simulink model "FlapDuuuuuragControlSimulatorForFriends"  (R2024b)
settings: Solver=VariableStepAuto  StartTime=0.0  StopTime=20  RelTol=1e-3
undefined symbols (not defined in the file): Asymptote, Body_Diameter, Body_Length, csv, DiscIntNeverNeededParam, Dragx, Dragy, Dry_Mass, Empty_Motor_Mass, Fin_Area, Flap_Length, Flap_width, flaps, Integral, Integral_Motor_Curve, Motorx, Motory, num_Flaps, optimize, Pressure, Propellent_Mass, Proportional, Rail_Angle, Temp, time_at_final, time_constants_to_final, wind_direction, wind_speed, wind_Z, Y_int_offset
libraries: simulink x4, simulink_extras x3, slpidlib x2, aerolibwind2 x2, aerolibutil x1, sharedtransform x1, eeGeneralControl x1
(part 1 of 2)
settings Model: PacingRate=10  Creator=jonse  LastModifiedBy=rjsoc
settings RTWCC: GPUComputeCapability=3.5

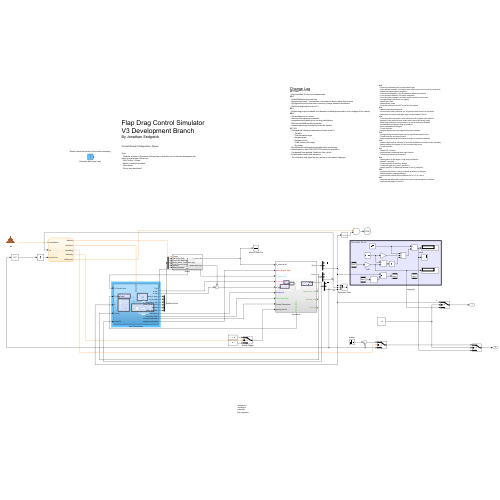
[thumbnail: Simulink's stored preview of the top-level diagram]
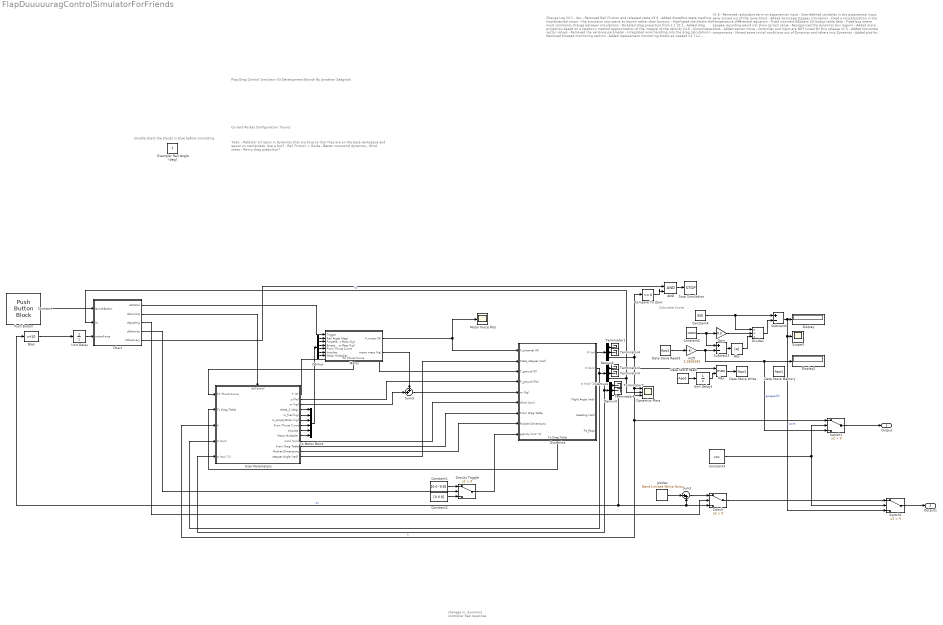
== system FlapDuuuuuragControlSimulatorForFriends ==
  note: changes in:
      |  dynamics
      | controller
      | flap response
  note: Todo:
      |  - Refactor all items in Dynamics that are blue so that they are on the base workspace and easier to manipulate. Use a bus?
      |  - Rail Friction + Guide
      |  - Better crosswind dynamics
      |  - Wind shear
      |  - Re-try drag prediction?
  note: Current Rocket Configuration: Taurus
  note: Double check the blocks in blue before simulating
  note: Calculate Score
  note: Flap Drag Control Simulator
      | V3 Development Branch
      | By Jonathan Sedgwick
  note: Change Log
      | V3.1 - dev
      | - Removed Rail Friction and releated state
      | V3.0
      | - Added Stateflow state machine
      | - Implemented motor - the simulator now starts at launch rather than burnout
      | - Highligted the blocks that most commonly change between simulations
      | - Disabled drag projection from 2.1
      | V2.1
      | - Added drag projection based on a Newton's method approximation of the integral of the velocity
      | V2.0
      | - Consolidated vector values
      | - Removed the variance parameter
      | - Integrated wind handling into the drag calculations
      | - Removed bloated monitoring section
      | - Added replacement monitoring blocks as needed
      | V1.7-L2
      | - Changed the following parameters to those of the L2
      | - Cd table
      | - Flap saturation angle
      | - Apogee target
      | - Apogee scoring
      | - Initial velocity and height
      | - Dry mass
      | - Re-defined the exponential input with better terminology
      | - Added option to use 2022-2023 CFD results for drag force
      | - Condensed User-defined Conditions into a block
      | - Added questionable wind equations
      | - The simulation now stops as soon as the all runs have hit apogee
  note: V1.6
      | - Removed redundant term on exponential input
      | - User-defined variables in the exponential input were moved out of the ramp block
      | - Added Simscape stepper simulation
      | - Fixed a miscalculation in the Temperature differential equation
      | - Fixed incorrect RASaero Cd lookup table data
      | - Fixed bug where apogee recording would not show correct value
      | - Reorganized the dynamics box (again)
      | - Added more plots
      | - Added sensor noise
      | - Controller and Input are NOT tuned for this release
      | V1.5
      | - Added horizontal components
      | - Moved some initial conditions out of Dynamics and others into Dynamics
      | - Added plot for velocity and flight angle (angle of attack? pitch?)
      | V1.4
      | - Fixed bug where simulation would end before all apogees were reached
      | - Apogee is now stored as max height rather than most recent height
      | - Body drag coefficient is now based on a lookup table from RASaero
      | - Incorperated post-apogee drag calculations
      | - More organizational changes
      | - Tuned controller
      | - Apogee displays are now organized by input condition
      | V1.3
      | - Changed from piecewise linear input to exponential input function
      | - Tuned controller and Input function
      | - Major oragnizational and formatting changes to increase readability
      | V1.2
      | - Added a high and low variance to the initial conditions to simulate motor variability
      | - Added displays for apogee in ft and corrosponding score
      | - Tuned controller
      | V1.1
      | - Added PID controller
      | - Implemented a saturated ramp input function
      | - Tuned input function and controller
      | V1.0
      | - Added effects of flap angle on flap drag contribution
      | - Added P controller
      | - Tuned controller to reach an altitude
      | - Combined graph for h and h_prediction
      | - Added graph for % difference between h and h_prediction
      | V0.2
      | - Implemented phisics 1 energy methods prediction for apogee
      | - Added graph for predicted apogee
      | - Implemented external initial conditions for h0, v0, m, and d
      | V0.1
      | - Implemented differential equations for motion and atmosphere conditions
      | - Implemented graphs of h and a
  AND : Logic  IconShape=distinctive  AllPortsSameDT=off  OutDataTypeStr=boolean
  Abs : Abs  SaturateOnIntegerOverflow=off
  Bias : Bias  Bias=10  SaturateOnIntegerOverflow=off
  Chart : Stateflow chart  TreatAsAtomicUnit=on
  Compare To Zero : simulink/Logic and Bit Operations/Compare To Zero  relop=<=  OutDataTypeStr=boolean
  Constant : Constant  Value=0
  Constant1 : Constant  Value=[0 0 -9.8]
  Constant2 : Constant  Value=[0 0 0]
  Constant3 : Constant  Value=csv
  Constant4 : Constant  Value=350
  Constant5 : Constant  Value=10000
  Data Store Read : DataStoreRead  DataStoreName=Apo1  IndexOptions=Index vector (dialog)  Indices=1  OutputSizes=1
  Data Store Read3 : DataStoreRead  DataStoreName=Apo1  IndexOptions=Index vector (dialog)  Indices=1  OutputSizes=1
  Data Store Write : DataStoreWrite  DataStoreName=Apo1  IndexOptions=Index vector (dialog)  Indices=1  OutputSizes=1
  Data Store Memory : DataStoreMemory  DataStoreName=Apo1  WriteAfterWriteMsg=warning  ShowAdditionalParam=off
  Demux : Demux  Outputs=6
  Demux1 : Demux  Outputs=3
  Demux2 : Demux  Outputs=3
  Demux4 : Demux  Outputs=3
  Display : Display
      settings: Format=bank
  Display2 : Display
      settings: Format=bank
  Divide1 : Product  Inputs=*/*
  Dynamics : Subsystem
      settings: PortSchema="{\"entries\":[{\"content\":{\"sides\":[{\"content\":{\"connectorIds\":[\"In1\",\"In2\",\"In3\",\"In4\",\"In5\",\"In6\",\"In7\",\"In8\",\"In9\"]},\"type\":\"ConnectorPlacement.EquallySpacedRectSide\",\"uuid\":\"61cf24c6-4793-46fb-bba1-f2879032278a\"},{\"content\":{\"connectorIds\":[\"Out1\",\"Out2\",\"Out3\",\"Out4\",\"Out5\",\"Out6\"],\"side\":\"RIGHT\"},\"type\":\"ConnectorPlacement.EquallySpacedRectSide\",\"uuid\":\"d36b1d95-1566-4e4d-8085-05406828bfee\"},{\"content\":{\"side\":\"TOP\"},\"type\":\"ConnectorPlacement.EquallySpacedRectSide\",\"uuid\":\"fa8074a3-9b0c-494d-b168-a3d8dc876f37\"},{\"content\":{\"connectorIds\":[\"Out7\"],\"side\":\"BOTTOM\"},\"type\":\"ConnectorPlacement.EquallySpacedRectSide\",\"uuid\":\"d0ccd591-4c20-4f19-a686-a0802005a38c\"}]},\"type\":\"ConnectorPlacement.EquallySpacedConnector\",\"uuid\":\"5370dd20-9b1c-4f64-993b-f7608f424fd6\"}],\"packageUris\":[\"http://schema.mathworks.com/mf0/Connector/R2020b\"],\"version\":\"1.0\"}"
  Dynamics Plots : Scope  NumInputPorts=3
  Example: Rail Angle (deg) : Constant  Value=7
  Gain : Gain  Gain=0.3
  Gravity Toggle : Switch  Criteria=u2 > Threshold  SaturateOnIntegerOverflow=off  InputSameDT=off
  Jostles : simulink/Sources/Band-Limited White Noise  Cov=[0.1]  Ts=0.1  seed=[23341]
  Max : MinMax  Function=max  Inputs=2  ZeroCross=off
  Motor : Subsystem
      settings: PortSchema="{\"entries\":[{\"content\":{\"sides\":[{\"content\":{\"connectorIds\":[\"In1\",\"In2\",\"In3\",\"In4\",\"In5\",\"In6\",\"In7\"]},\"type\":\"ConnectorPlacement.EquallySpacedRectSide\",\"uuid\":\"6892474e-c13b-4b5d-a78a-550e13a4fcf7\"},{\"content\":{\"connectorIds\":[\"Out1\",\"Out2\"],\"side\":\"RIGHT\"},\"type\":\"ConnectorPlacement.EquallySpacedRectSide\",\"uuid\":\"18cd9a73-be62-415c-a5c9-b5315f96bd44\"},{\"content\":{\"side\":\"TOP\"},\"type\":\"ConnectorPlacement.EquallySpacedRectSide\",\"uuid\":\"19941a30-b527-4a81-9ce0-74fdb4c32049\"},{\"content\":{\"connectorIds\":[\"Out3\"],\"side\":\"BOTTOM\"},\"type\":\"ConnectorPlacement.EquallySpacedRectSide\",\"uuid\":\"d47e24a6-a8af-4693-b00f-f9087fef628a\"}]},\"type\":\"ConnectorPlacement.EquallySpacedConnector\",\"uuid\":\"0b620e34-0fcb-46c3-97c7-1b93d7cb0d0f\"}],\"packageUris\":[\"http://schema.mathworks.com/mf0/Connector/R2020b\"],\"version\":\"1.0\"}"
  Motor Force Plot : Scope
  Push Button : PushButtonBlock  ButtonText=Launch  Icon=Triangle  IconAlignment=Top  IconColor=On  OffValue=0.000000
  Scope3 : Scope
  Stop Simulation : Stop
  Subtract2 : Sum  Inputs=+-
  Subtract3 : Sum  Inputs=+-
  Sum1 : Sum  Inputs=|++
  Sum3 : Sum  Inputs=++|
  Switch : Switch  Criteria=u2 > Threshold  SaturateOnIntegerOverflow=off  InputSameDT=off
  Switch1 : Switch  Criteria=u2 > Threshold  SaturateOnIntegerOverflow=off  InputSameDT=off
  Switch2 : Switch  Criteria=u2 > Threshold  SaturateOnIntegerOverflow=off  InputSameDT=off
  Terminator{1..4,7..8} (6 alike) : Terminator
  To Motor Block : BusCreator  Inputs=6
  Unit Delay : UnitDelay  SampleTime=-1  HasFrameUpgradeWarning=on
  Unit Delay1 : UnitDelay  SampleTime=-1  HasFrameUpgradeWarning=on
  User Parameters : Subsystem
      settings: PortSchema="{\"entries\":[{\"content\":{\"sides\":[{\"content\":{\"connectorIds\":[\"In1\",\"In2\",\"In3\",\"In4\",\"In5\"]},\"type\":\"ConnectorPlacement.EquallySpacedRectSide\",\"uuid\":\"67ceafc0-d2dd-45da-bafe-c1e73a1e832c\"},{\"content\":{\"connectorIds\":[\"Out1\",\"Out2\",\"Out3\",\"Out4\",\"Out5\",\"Out6\",\"Out7\",\"Out8\",\"Out9\",\"Out10\",\"Out11\",\"Out12\",\"Out13\"],\"side\":\"RIGHT\"},\"type\":\"ConnectorPlacement.EquallySpacedRectSide\",\"uuid\":\"fdcb3816-6022-4f62-9865-dec1f25bccbe\"},{\"content\":{\"connectorIds\":[\"In6\"],\"side\":\"TOP\"},\"type\":\"ConnectorPlacement.EquallySpacedRectSide\",\"uuid\":\"c0a2d968-8bba-41a7-998d-7d8e966bd078\"}]},\"type\":\"ConnectorPlacement.EquallySpacedConnector\",\"uuid\":\"e02f46ef-3454-4fc3-b120-1dd0bd81dbda\"}],\"packageUris\":[\"http://schema.mathworks.com/mf0/Connector/R2020b\"],\"version\":\"1.0\"}"
  m2ft : Gain  Gain=3.2808399
  Output : Outport
  Output1 : Outport  Port=2
  wires:
  Chart/1(doMotor) -> Motor/1(Trigger)
  Constant/1 -> Chart/1(launchButton)
  Demux1/2 -> Terminator3/1
  Demux1/1 -> Terminator2/1
  Demux1/3 -> Chart/2(Vz), Dynamics Plots/2  "Vz"
  Demux2/1 -> Terminator1/1
  Demux2/2 -> Terminator4/1
  Dynamics/1(R (m)) -> Demux2/1
  Dynamics/2(V (m/s)) -> User Parameters/4(V (m/s)), Demux1/1
  Chart/2(doControl) -> User Parameters/6(doControl)
  User Parameters/10(wind (m/s)) -> Dynamics/6(Wind (m/s))
  Motor/2(motor mass (kg)) -> Sum3/1
  Sum3/1 -> Dynamics/5(m (kg))
  Constant1/1 -> Gravity Toggle/1
  Chart/4(doGravity) -> Gravity Toggle/2
  Constant2/1 -> Gravity Toggle/3
  Gravity Toggle/1 -> Dynamics/9(gravity (m/s^2))
  Unit Delay/1 -> Chart/3(motorForce)
  Chart/5(inRecovery) -> AND/1
  Compare To Zero/1 -> AND/2
  AND/1 -> Stop Simulation/1
  Subtract3/1 -> Abs/1
  Abs/1 -> Divide1/3
  Constant4/1 -> Subtract2/1, Divide1/1
  Subtract2/1 -> Switch2/3, Scope3/1, Display/1  "score"
  Divide1/1 -> Subtract2/2
  Gain/1 -> Divide1/2
  Constant5/1 -> Subtract3/1, Gain/1
  m2ft/1 -> Switch1/3, Display2/1, Subtract3/2  "apogee(ft)"
  Data Store Read/1 -> Unit Delay1/1
  Max/1 -> Data Store Write/1
  Unit Delay1/1 -> Max/2
  Data Store Read3/1 -> m2ft/1
  Demux2/3 -> Compare To Zero/1, User Parameters/3(h), Switch1/1, Dynamics Plots/1, Max/1  "h"
  Demux4/1 -> Terminator7/1
  Dynamics/3(a (m/s^2)) -> User Parameters/5(a (m/s^2)), Demux4/1
  Demux4/3 -> Bias/1, Sum1/2, Switch/3, Dynamics Plots/3  "az"
  Demux4/2 -> Terminator8/1
  Sum1/1 -> Switch/1
  Chart/3(doJostling) -> Switch/2
  Jostles/1 -> Sum1/1
  Switch/1 -> Switch2/1
  Bias/1 -> Unit Delay/1
  Motor/1(F_motor (N)) -> Dynamics/1(F_external (N)), Motor Force Plot/1
  User Parameters/1(T (K)) -> Dynamics/3(T_ground (K))
  User Parameters/2(p (Pa)) -> Dynamics/4(P_ground (Pa))
  User Parameters/3(m (kg)) -> Sum3/2
  Motor/3(To Thrust Curve) -> User Parameters/1(To Thrust Curve)
  User Parameters/5(m_fuel (kg)) -> To Motor Block/2
  User Parameters/6(m_emptyMotor (kg)) -> To Motor Block/3
  User Parameters/7(From Thrust Curve) -> To Motor Block/4
  User Parameters/8(Impulse) -> To Motor Block/5
  User Parameters/9(Motor Multiplier) -> To Motor Block/6
  User Parameters/4(theta_0 (deg)) -> To Motor Block/1
  To Motor Block/1 -> Demux/1
  Demux/6 -> Motor/7(Motor Multiplier)
  Demux/5 -> Motor/6(Impulse)
  Demux/4 -> Motor/5(From Thrust Curve)
  Demux/3 -> Motor/4(Empty Motor Case Mass (kg))
  Demux/2 -> Motor/3(Propellent Mass (kg))
  Demux/1 -> Motor/2(Rail Angle (deg))
  User Parameters/11(From Drag Table) -> Dynamics/7(From Drag Table)
  Dynamics/7(To Drag Table) -> User Parameters/2(To Drag Table)
  User Parameters/12(Rocket Dimensions) -> Dynamics/8(Rocket Dimensions)
  User Parameters/13(stepper Angle (rad)) -> Dynamics/2(theta_stepper (rad))
  Switch1/1 -> Output/1
  Switch2/1 -> Output1/1
  Constant3/1 -> Switch1/2, Switch2/2

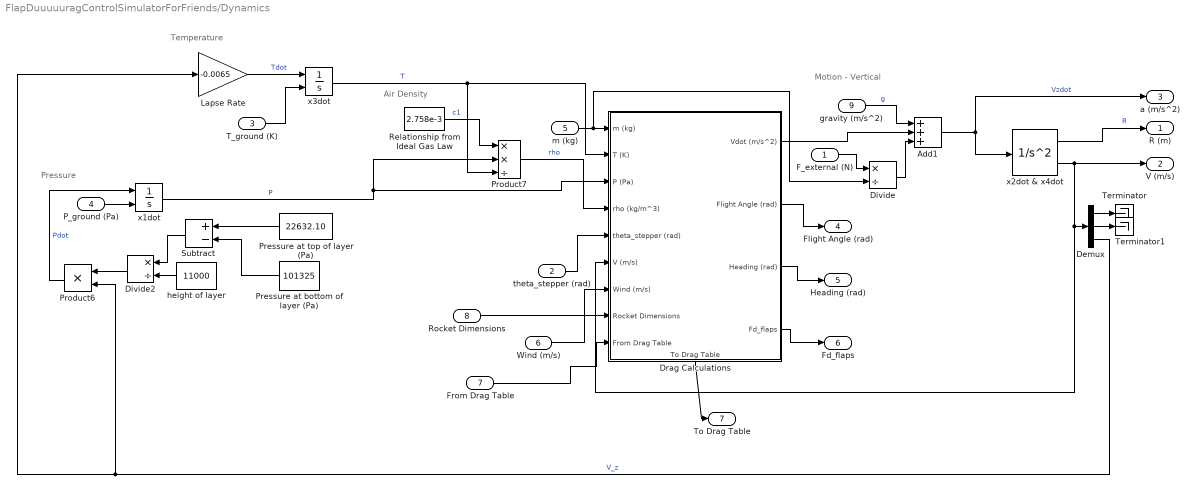
== system FlapDuuuuuragControlSimulatorForFriends/Dynamics ==
  note: Motion - Vertical
  note: Temperature
  note: Pressure
  note: Air Density
  F_external (N) : Inport
  theta_stepper (rad) : Inport  Port=2
  T_ground (K) : Inport  Port=3
  P_ground (Pa) : Inport  Port=4
  m (kg) : Inport  Port=5
  Wind (m/s) : Inport  Port=6
  From Drag Table : Inport  Port=7
  Rocket Dimensions : Inport  Port=8
  gravity (m/s^2) : Inport  Port=9
  Add1 : Sum  Inputs=+++
  Demux : Demux  Outputs=3
  Divide : Product  Inputs=*/
  Divide2 : Product  Inputs=*/
  Drag Calculations : Subsystem  Variant=on  VariantControlMode=label  VariantControl=Subsystem  LabelModeActiveChoice=RASaero Lookup
      settings: PortSchema="{\"entries\":[{\"content\":{\"sides\":[{\"content\":{\"connectorIds\":[\"In1\",\"In2\",\"In3\",\"In4\",\"In5\",\"In6\",\"In7\",\"In8\",\"In9\"]},\"type\":\"ConnectorPlacement.EquallySpacedRectSide\",\"uuid\":\"9dd66c9f-8665-4301-bc82-0ebfb6103ae4\"},{\"content\":{\"connectorIds\":[\"Out1\",\"Out2\",\"Out3\",\"Out4\"],\"side\":\"RIGHT\"},\"type\":\"ConnectorPlacement.EquallySpacedRectSide\",\"uuid\":\"50f6fdcb-0f1b-4884-96dd-6344c1c927c9\"},{\"content\":{\"side\":\"TOP\"},\"type\":\"ConnectorPlacement.EquallySpacedRectSide\",\"uuid\":\"6972989e-5f03-41b6-a7d3-55bb73d6efee\"},{\"content\":{\"connectorIds\":[\"Out5\"],\"side\":\"BOTTOM\"},\"type\":\"ConnectorPlacement.EquallySpacedRectSide\",\"uuid\":\"84fc1c4d-1e1e-4679-8051-8a9b135287a7\"}]},\"type\":\"ConnectorPlacement.EquallySpacedConnector\",\"uuid\":\"59c584d9-fea7-42d3-821f-ecefb9356ae6\"}],\"packageUris\":[\"http://schema.mathworks.com/mf0/Connector/R2020b\"],\"version\":\"1.0\"}"
  Lapse Rate : Gain  Gain=-0.0065
  Pressure at bottom of layer (Pa) : Constant  Value=101325
  Pressure at top of layer (Pa) : Constant  Value=22632.10
  Product6 : Product
  Product7 : Product  Inputs=**/
  Relationship from Ideal Gas Law : Constant  Value=2.758e-3
  Subtract : Sum  Inputs=+-
  Terminator : Terminator
  Terminator1 : Terminator
  height of layer : Constant  Value=11000
  x1dot : Integrator  InitialConditionSource=external  InitialCondition=81495.52
  x2dot & x4dot : SecondOrderIntegrator
  x3dot : Integrator  InitialConditionSource=external  InitialCondition=18.4 + 237.15
  R (m) : Outport
  V (m/s) : Outport  Port=2
  a (m/s^2) : Outport  Port=3
  Flight Angle (rad) : Outport  Port=4
  Heading (rad) : Outport  Port=5
  Fd_flaps : Outport  Port=6
  To Drag Table : Outport  Port=7
  wires:
  x2dot & x4dot/1 -> R (m)/1  "R"
  Add1/1 -> x2dot & x4dot/1, a (m/s^2)/1  "Vzdot"
  Demux/3 -> Product6/2, Lapse Rate/1  "V_z"
  Divide2/1 -> Product6/1
  gravity (m/s^2)/1 -> Add1/1  "g"
  Lapse Rate/1 -> x3dot/1  "Tdot"
  Product6/1 -> x1dot/1  "Pdot"
  Pressure at top of layer (Pa)/1 -> Subtract/1
  height of layer/1 -> Divide2/2
  Pressure at bottom of layer (Pa)/1 -> Subtract/2
  Subtract/1 -> Divide2/1
  P_ground (Pa)/1 -> x1dot/2
  T_ground (K)/1 -> x3dot/2
  m (kg)/1 -> Divide/2, Drag Calculations/1(m (kg))
  theta_stepper (rad)/1 -> Drag Calculations/5(theta_stepper (rad))
  Drag Calculations/1(Vdot (m/s^2)) -> Add1/2
  Drag Calculations/2(Flight Angle (rad)) -> Flight Angle (rad)/1
  Drag Calculations/3(Heading (rad)) -> Heading (rad)/1
  Product7/1 -> Drag Calculations/4(rho (kg/m^3))  "rho"
  Relationship from Ideal Gas Law/1 -> Product7/1  "c1"
  x1dot/1 -> Product7/2, Drag Calculations/3(P (Pa))  "P"
  x3dot/1 -> Drag Calculations/2(T (K)), Product7/3  "T"
  Wind (m/s)/1 -> Drag Calculations/7(Wind (m/s))
  x2dot & x4dot/2 -> Drag Calculations/6(V (m/s)), Demux/1, V (m/s)/1
  Demux/2 -> Terminator1/1
  Demux/1 -> Terminator/1
  Drag Calculations/4(Fd_flaps) -> Fd_flaps/1
  Divide/1 -> Add1/3
  F_external (N)/1 -> Divide/1
  Drag Calculations/5(To Drag Table) -> To Drag Table/1
  From Drag Table/1 -> Drag Calculations/9(From Drag Table)
  Rocket Dimensions/1 -> Drag Calculations/8(Rocket Dimensions)

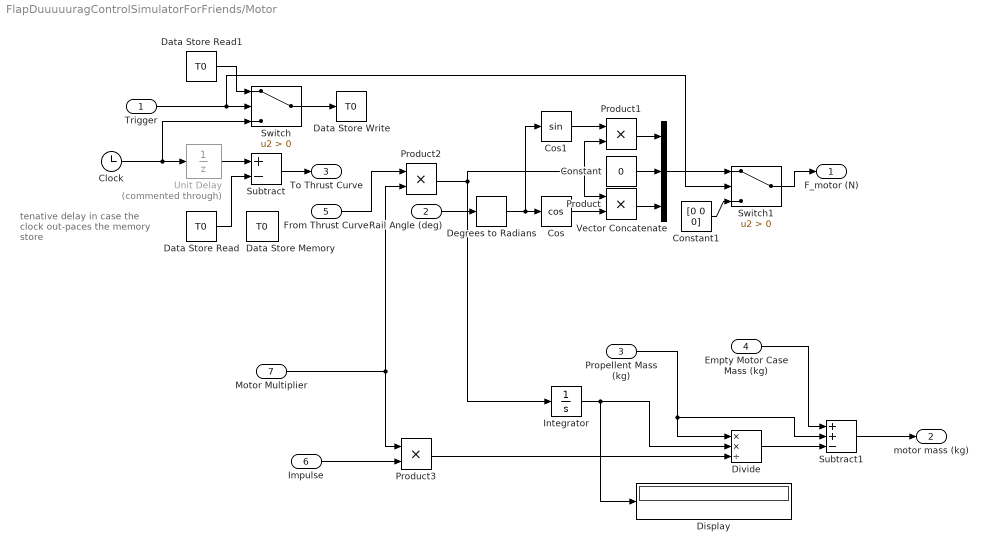
== system FlapDuuuuuragControlSimulatorForFriends/Motor ==
  note: tenative delay in case the clock out-paces the memory store
  Trigger : Inport
  Rail Angle (deg) : Inport  Port=2
  Propellent Mass (kg) : Inport  Port=3
  Empty Motor Case Mass (kg) : Inport  Port=4
  From Thrust Curve : Inport  Port=5
  Impulse : Inport  Port=6
  Motor Multiplier : Inport  Port=7
  Clock : Clock
  Constant : Constant  Value=0
  Constant1 : Constant  Value=[0 0 0]
  Cos : Trigonometry  Operator=cos
  Cos1 : Trigonometry
  Data Store Memory : DataStoreMemory  DataStoreName=T0  WriteAfterWriteMsg=warning  ShowAdditionalParam=off
  Data Store Read : DataStoreRead  DataStoreName=T0  IndexOptions=Index vector (dialog)  Indices=1  OutputSizes=1
  Data Store Read1 : DataStoreRead  DataStoreName=T0  IndexOptions=Index vector (dialog)  Indices=1  OutputSizes=1
  Data Store Write : DataStoreWrite  DataStoreName=T0  IndexOptions=Index vector (dialog)  Indices=1  OutputSizes=1
  Degrees to Radians : simulink_extras/Transformations/Degrees to Radians
  Display : Display
      settings: Format=long_e
  Divide : Product  Inputs=**/
  Integrator : Integrator
  Product{,1..3} (4 alike) : Product
  Subtract : Sum  Inputs=+-
  Subtract1 : Sum  Inputs=++-
  Switch : Switch  Criteria=u2 > Threshold  SaturateOnIntegerOverflow=off  InputSameDT=off
  Switch1 : Switch  Criteria=u2 > Threshold  SaturateOnIntegerOverflow=off  InputSameDT=off
  Unit Delay : UnitDelay  Commented=through  SampleTime=-1  HasFrameUpgradeWarning=on
  Vector Concatenate : Concatenate  NumInputs=3
  F_motor (N) : Outport
  motor mass (kg) : Outport  Port=2
  To Thrust Curve : Outport  Port=3
  wires:
  Clock/1 -> Unit Delay/1, Switch/3
  Product2/1 -> Product/1, Product1/2, Integrator/1
  Subtract/1 -> To Thrust Curve/1
  Switch/1 -> Data Store Write/1
  Data Store Read/1 -> Subtract/2
  Data Store Read1/1 -> Switch/1
  Trigger/1 -> Switch1/2, Switch/2
  Rail Angle (deg)/1 -> Degrees to Radians/1
  Degrees to Radians/1 -> Cos1/1, Cos/1
  Constant/1 -> Vector Concatenate/2
  Vector Concatenate/1 -> Switch1/1
  Cos1/1 -> Product1/1
  Cos/1 -> Product/2
  Product1/1 -> Vector Concatenate/1
  Product/1 -> Vector Concatenate/3
  Unit Delay/1 -> Subtract/1
  Integrator/1 -> Display/1, Divide/2
  Divide/1 -> Subtract1/3
  Switch1/1 -> F_motor (N)/1
  Constant1/1 -> Switch1/3
  Product3/1 -> Divide/3
  From Thrust Curve/1 -> Product2/1
  Empty Motor Case Mass (kg)/1 -> Subtract1/1
  Propellent Mass (kg)/1 -> Subtract1/2, Divide/1
  Impulse/1 -> Product3/2
  Motor Multiplier/1 -> Product2/2, Product3/1
  Subtract1/1 -> motor mass (kg)/1

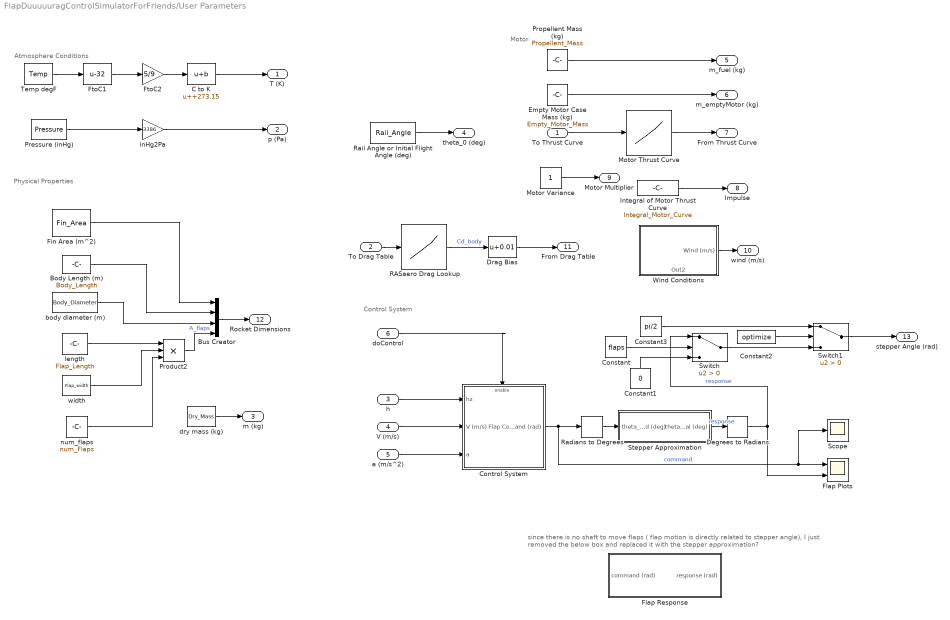
== system FlapDuuuuuragControlSimulatorForFriends/User Parameters ==
  note: since there is no shaft to move flaps ( flap motion is directly related to stepper angle), I just removed the below box and replaced it with the stepper approximation?
  note: Control System
  note: Physical Properties
  note: Motor
  note: Atmosphere Conditions
  To Thrust Curve : Inport
  To Drag Table : Inport  Port=2
  h : Inport  Port=3
  V (m/s) : Inport  Port=4
  a (m/s^2) : Inport  Port=5
  doControl : Inport  Port=6
  Body Length (m) : Constant  Value=Body_Length
  Bus Creator : BusCreator  Inputs=4
  C to K : Bias  Bias=+273.15  SaturateOnIntegerOverflow=off
  Constant : Constant  Value=flaps
  Constant1 : Constant  Value=0
  Constant2 : Constant  Value=optimize
  Constant3 : Constant  Value=pi/2
  Control System : Subsystem  TreatAsAtomicUnit=on
  Degrees to Radians : simulink_extras/Transformations/Degrees to Radians
  Drag Bias : Bias  Bias=0.01  SaturateOnIntegerOverflow=off
  Empty Motor Case Mass (kg) : Constant  Value=Empty_Motor_Mass
  Fin Area (m^2) : Constant  Value=Fin_Area
  Flap Plots : Scope  NumInputPorts=2
  Flap Response : Subsystem
  FtoC1 : Bias  Bias=-32  SaturateOnIntegerOverflow=off
  FtoC2 : Gain  Gain=5/9
  Integral of Motor Thrust Curve : Constant  Value=Integral_Motor_Curve
  Motor Thrust Curve : Lookup_n-D  NumberOfTableDimensions=1  BreakpointsForDimension1=Motory  BeginIndexSearchUsingPreviousIndexResult=on  Table=Motorx  RemoveProtectionInput=on  InternalRulePriority=Speed  RndMeth=Simplest
  Motor Variance : Constant
  Pressure (inHg) : Constant  Value=Pressure
  Product2 : Product  Inputs=3
  Propellent Mass (kg) : Constant  Value=Propellent_Mass
  RASaero Drag Lookup : Lookup_n-D  NumberOfTableDimensions=1  BreakpointsForDimension1=Dragy  Table=Dragx  InternalRulePriority=Speed  RndMeth=Simplest
  Radians to Degrees : simulink_extras/Transformations/Radians to Degrees
  Rail Angle or Initial Flight Angle (deg) : Constant  Value=Rail_Angle
  Scope : Scope
  Stepper Approximation : Subsystem
  Switch : Switch  Criteria=u2 > Threshold  SaturateOnIntegerOverflow=off  InputSameDT=off
  Switch1 : Switch  Criteria=u2 > Threshold  SaturateOnIntegerOverflow=off  InputSameDT=off
  Temp degF : Constant  Value=Temp
  Wind Conditions : Subsystem  Variant=on  VariantControlMode=label  VariantControl=Wind Conditions  LabelModeActiveChoice=Wind Conditions
      settings: PortSchema="{\"entries\":[{\"content\":{\"sides\":[{\"content\":{},\"type\":\"ConnectorPlacement.EquallySpacedRectSide\",\"uuid\":\"35ea3996-9f39-4348-a2f7-6673d7935930\"},{\"content\":{\"connectorIds\":[\"Out1\"],\"side\":\"RIGHT\"},\"type\":\"ConnectorPlacement.EquallySpacedRectSide\",\"uuid\":\"94fd4444-0f85-409c-9171-39c8ab598537\"},{\"content\":{\"side\":\"TOP\"},\"type\":\"ConnectorPlacement.EquallySpacedRectSide\",\"uuid\":\"62448ab5-3199-44a8-971b-c852add313d4\"},{\"content\":{\"connectorIds\":[\"Out2\"],\"side\":\"BOTTOM\"},\"type\":\"ConnectorPlacement.EquallySpacedRectSide\",\"uuid\":\"cebe46ea-63f9-4a79-8119-dacf57e6cf90\"}]},\"type\":\"ConnectorPlacement.EquallySpacedConnector\",\"uuid\":\"bdaf23a0-a7d0-496f-94c8-d1d69587b918\"}],\"packageUris\":[\"http://schema.mathworks.com/mf0/Connector/R2020b\"],\"version\":\"1.0\"}"
  body diameter (m) : Constant  Value=Body_Diameter
  dry mass (kg) : Constant  Value=Dry_Mass
  inHg2Pa : Gain  Gain=3386
  length : Constant  Value=Flap_Length
  num_flaps : Constant  Value=num_Flaps
  width : Constant  Value=Flap_width
  T (K) : Outport
  p (Pa) : Outport  Port=2
  m (kg) : Outport  Port=3
  theta_0 (deg) : Outport  Port=4
  m_fuel (kg) : Outport  Port=5
  m_emptyMotor (kg) : Outport  Port=6
  From Thrust Curve : Outport  Port=7
  Impulse : Outport  Port=8
  Motor Multiplier : Outport  Port=9
  wind (m/s) : Outport  Port=10
  From Drag Table : Outport  Port=11
  Rocket Dimensions : Outport  Port=12
  stepper Angle (rad) : Outport  Port=13
  wires:
  dry mass (kg)/1 -> m (kg)/1
  Pressure (inHg)/1 -> inHg2Pa/1
  C to K/1 -> T (K)/1
  Rail Angle or Initial Flight Angle (deg)/1 -> theta_0 (deg)/1
  Temp degF/1 -> FtoC1/1
  inHg2Pa/1 -> p (Pa)/1
  FtoC2/1 -> C to K/1
  FtoC1/1 -> FtoC2/1
  Propellent Mass (kg)/1 -> m_fuel (kg)/1
  Empty Motor Case Mass (kg)/1 -> m_emptyMotor (kg)/1
  To Thrust Curve/1 -> Motor Thrust Curve/1
  Motor Thrust Curve/1 -> From Thrust Curve/1
  Integral of Motor Thrust Curve/1 -> Impulse/1
  Motor Variance/1 -> Motor Multiplier/1
  Wind Conditions/1(Wind (m/s)) -> wind (m/s)/1
  Drag Bias/1 -> From Drag Table/1
  RASaero Drag Lookup/1 -> Drag Bias/1  "Cd_body"
  To Drag Table/1 -> RASaero Drag Lookup/1
  length/1 -> Product2/1
  width/1 -> Product2/2
  num_flaps/1 -> Product2/3
  Product2/1 -> Bus Creator/4  "A_flaps"
  Fin Area (m^2)/1 -> Bus Creator/1
  Body Length (m)/1 -> Bus Creator/2
  body diameter (m)/1 -> Bus Creator/3
  Bus Creator/1 -> Rocket Dimensions/1
  Degrees to Radians/1 -> Flap Plots/2, Switch/1  "response"
  Control System/1(Flap Command (rad)) -> Scope/1, Flap Plots/1, Radians to Degrees/1  "command"
  doControl/1 -> Control System/Enable
  a (m/s^2)/1 -> Control System/3(a)
  V (m/s)/1 -> Control System/2(V (m/s))
  h/1 -> Control System/1(hz)
  Constant/1 -> Switch/2
  Switch/1 -> Switch1/3
  Constant1/1 -> Switch/3
  Constant2/1 -> Switch1/2
  Constant3/1 -> Switch1/1
  Switch1/1 -> stepper Angle (rad)/1
  Radians to Degrees/1 -> Stepper Approximation/1(theta_desired (deg))
  Stepper Approximation/1(theta_actual (deg)) -> Degrees to Radians/1  "response"

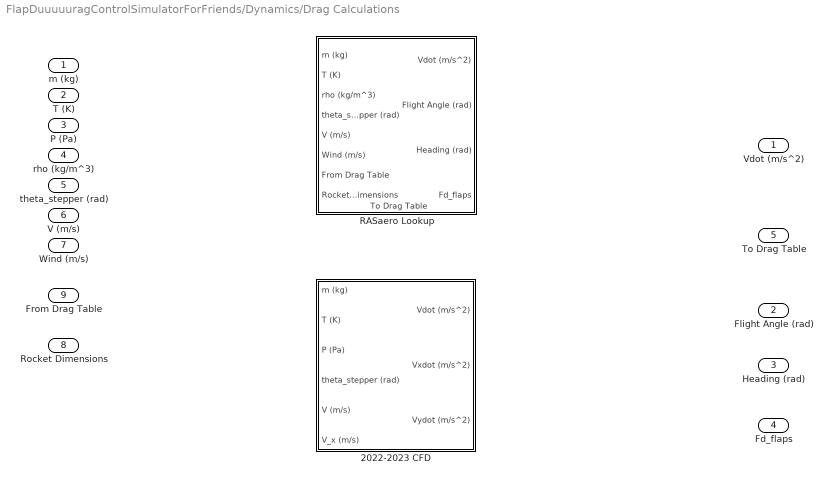
== system FlapDuuuuuragControlSimulatorForFriends/Dynamics/Drag Calculations ==
  m (kg) : Inport
  T (K) : Inport  Port=2
  P (Pa) : Inport  Port=3
  rho (kg/m^3) : Inport  Port=4
  theta_stepper (rad) : Inport  Port=5
  V (m/s) : Inport  Port=6
  Wind (m/s) : Inport  Port=7
  Rocket Dimensions : Inport  Port=8
  From Drag Table : Inport  Port=9
  2022-2023 CFD : Subsystem  VariantControl=2022-2023 CFD
  RASaero Lookup : Subsystem  VariantControl=RASaero Lookup
      settings: PortSchema="{\"entries\":[{\"content\":{\"sides\":[{\"content\":{\"connectorIds\":[\"In1\",\"In2\",\"In3\",\"In4\",\"In5\",\"In6\",\"In7\",\"In8\"]},\"type\":\"ConnectorPlacement.EquallySpacedRectSide\",\"uuid\":\"9dd66c9f-8665-4301-bc82-0ebfb6103ae4\"},{\"content\":{\"connectorIds\":[\"Out1\",\"Out2\",\"Out3\",\"Out4\"],\"side\":\"RIGHT\"},\"type\":\"ConnectorPlacement.EquallySpacedRectSide\",\"uuid\":\"50f6fdcb-0f1b-4884-96dd-6344c1c927c9\"},{\"content\":{\"side\":\"TOP\"},\"type\":\"ConnectorPlacement.EquallySpacedRectSide\",\"uuid\":\"6972989e-5f03-41b6-a7d3-55bb73d6efee\"},{\"content\":{\"connectorIds\":[\"Out5\"],\"side\":\"BOTTOM\"},\"type\":\"ConnectorPlacement.EquallySpacedRectSide\",\"uuid\":\"618f21cc-2a79-4282-bd76-51c29f61df59\"}]},\"type\":\"ConnectorPlacement.EquallySpacedConnector\",\"uuid\":\"59c584d9-fea7-42d3-821f-ecefb9356ae6\"}],\"packageUris\":[\"http://schema.mathworks.com/mf0/Connector/R2020b\"],\"version\":\"1.0\"}"
  Vdot (m/s^2) : Outport
  Flight Angle (rad) : Outport  Port=2
  Heading (rad) : Outport  Port=3
  Fd_flaps : Outport  Port=4
  To Drag Table : Outport  Port=5

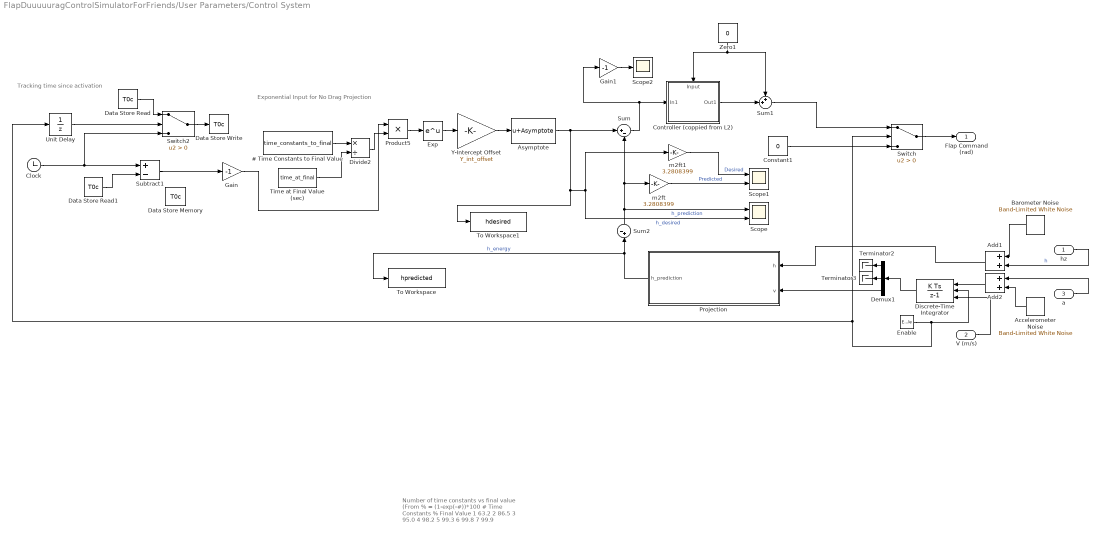
== system FlapDuuuuuragControlSimulatorForFriends/User Parameters/Control System ==
  note: Tracking time since activation
  note: Exponential Input for No Drag Projection
  note: Number of time constants vs final value
      | (From % = (1-exp(-#))*100
      |
      | # Time Constants
      | % Final Value
      |
      | 1
      | 63.2
      |
      | 2
      | 86.5
      |
      | 3
      | 95.0
      |
      | 4
      | 98.2
      |
      | 5
      | 99.3
      |
      | 6
      | 99.8
      |
      | 7
      | 99.9
  hz : Inport
  V (m/s) : Inport  Port=2
  a : Inport  Port=3
  Enable : EnablePort  ShowOutputPort=on
  # Time Constants to Final Value : Constant  Value=time_constants_to_final
  Accelerometer Noise : simulink/Sources/Band-Limited White Noise  Cov=[0.01]  Ts=0.01  seed=[23342]
  Add1 : Sum
  Add2 : Sum
  Asymptote : Bias  Bias=Asymptote  SaturateOnIntegerOverflow=off
  Barometer Noise : simulink/Sources/Band-Limited White Noise  Cov=[0.01]  Ts=0.01  seed=[23341]
  Clock : Clock
  Constant1 : Constant  Value=0
  Controller (coppied from L2) : Subsystem  Variant=on
      settings: PortSchema="{\"entries\":[{\"content\":{\"sides\":[{\"content\":{\"connectorIds\":[\"In1\"]},\"type\":\"ConnectorPlacement.EquallySpacedRectSide\",\"uuid\":\"1d14b0ba-faa0-4321-b836-d968053f0108\"},{\"content\":{\"connectorIds\":[\"Out1\"],\"side\":\"RIGHT\"},\"type\":\"ConnectorPlacement.EquallySpacedRectSide\",\"uuid\":\"8637ad70-7bf6-4cc6-9fdf-243ab9d315bc\"},{\"content\":{\"connectorIds\":[\"In2\"],\"side\":\"TOP\"},\"type\":\"ConnectorPlacement.EquallySpacedRectSide\",\"uuid\":\"091fa34f-5366-4b1d-b288-d7c22d23e803\"}]},\"type\":\"ConnectorPlacement.EquallySpacedConnector\",\"uuid\":\"7981e116-3e12-4e46-be74-9cbcc964a4cc\"}],\"packageUris\":[\"http://schema.mathworks.com/mf0/Connector/R2020b\"],\"version\":\"1.0\"}"
  Data Store Memory : DataStoreMemory  DataStoreName=T0c  WriteAfterWriteMsg=warning  ShowAdditionalParam=off
  Data Store Read : DataStoreRead  DataStoreName=T0c  IndexOptions=Index vector (dialog)  Indices=1  OutputSizes=1
  Data Store Read1 : DataStoreRead  DataStoreName=T0c  IndexOptions=Index vector (dialog)  Indices=1  OutputSizes=1
  Data Store Write : DataStoreWrite  DataStoreName=T0c  IndexOptions=Index vector (dialog)  Indices=1  OutputSizes=1
  Demux1 : Demux  Outputs=3
  Discrete-Time Integrator : DiscreteIntegrator  ExternalReset=rising  InitialConditionSource=external  InitialCondition=302.3616  SampleTime=0.01  ICPrevOutput=DiscIntNeverNeededParam  ICPrevScaledInput=DiscIntNeverNeededParam
  Divide2 : Product  Inputs=*/
  Exp : Math
  Gain : Gain  Gain=-1
  Gain1 : Gain  Gain=-1
  Product5 : Product
  Projection : Subsystem
  Scope : Scope  NumInputPorts=2
  Scope1 : Scope  NumInputPorts=2
  Scope2 : Scope
  Subtract1 : Sum  Inputs=+-
  Sum : Sum  Inputs=|+-
  Sum1 : Sum  Inputs=++|
  Sum2 : Sum  Inputs=-+|
  Switch : Switch  Criteria=u2 > Threshold  SaturateOnIntegerOverflow=off  InputSameDT=off
  Switch2 : Switch  Criteria=u2 > Threshold  SaturateOnIntegerOverflow=off  InputSameDT=off
  Terminator2 : Terminator
  Terminator3 : Terminator
  Time at Final Value (sec) : Constant  Value=time_at_final
  To Workspace : ToWorkspace  VariableName=hpredicted  SaveFormat=Timeseries  SampleTime=-1
  To Workspace1 : ToWorkspace  VariableName=hdesired  SaveFormat=Timeseries  SampleTime=-1
  Unit Delay : UnitDelay  SampleTime=-1  HasFrameUpgradeWarning=on
  Y-Intercept Offset : Gain  Gain=Y_int_offset
  Zero1 : Constant  Value=0  OutDataTypeStr=Inherit: Inherit via back propagation
  m2ft : Gain  Gain=3.2808399
  m2ft1 : Gain  Gain=3.2808399
  Flap Command (rad) : Outport
  wires:
  Sum/1 -> Gain1/1, Controller (coppied from L2)/1(In1)
  Demux1/2 -> Terminator3/1
  Demux1/1 -> Terminator2/1
  Time at Final Value (sec)/1 -> Divide2/2
  Accelerometer Noise/1 -> Add2/2
  Exp/1 -> Y-Intercept Offset/1
  Projection/1(h_prediction) -> Sum2/2, To Workspace/1  "h_energy"
  Controller (coppied from L2)/1(Out1) -> Sum1/2
  a/1 -> Add2/1
  Add2/1 -> Discrete-Time Integrator/1
  Zero1/1 -> Sum1/1, Controller (coppied from L2)/2(Input)
  Barometer Noise/1 -> Add1/1
  Add1/1 -> Projection/1(h)
  Sum1/1 -> Switch/1
  Discrete-Time Integrator/1 -> Demux1/1
  hz/1 -> Add1/2  "h"
  Demux1/3 -> Projection/2(v)
  Divide2/1 -> Product5/2
  Sum2/1 -> Sum/2, m2ft/1, Scope/1  "h_prediction"
  Asymptote/1 -> Sum/1, To Workspace1/1, m2ft1/1, Scope/2  "h_desired"
  Y-Intercept Offset/1 -> Asymptote/1
  Product5/1 -> Exp/1
  # Time Constants to Final Value/1 -> Divide2/1
  Constant1/1 -> Switch/3
  Switch/1 -> Flap Command (rad)/1
  V (m/s)/1 -> Discrete-Time Integrator/3
  Gain/1 -> Product5/1
  Switch2/1 -> Data Store Write/1
  Clock/1 -> Subtract1/1, Switch2/3
  Enable/1 -> Discrete-Time Integrator/2, Unit Delay/1, Switch/2
  Data Store Read/1 -> Switch2/1
  Data Store Read1/1 -> Subtract1/2
  Subtract1/1 -> Gain/1
  Unit Delay/1 -> Switch2/2
  Gain1/1 -> Scope2/1
  m2ft/1 -> Scope1/2  "Predicted"
  m2ft1/1 -> Scope1/1  "Desired"

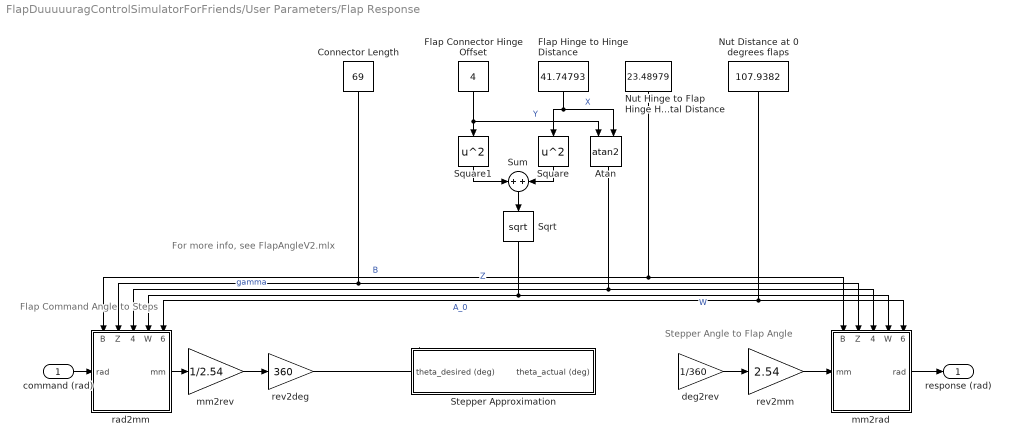
== system FlapDuuuuuragControlSimulatorForFriends/User Parameters/Flap Response ==
  note: For more info, see FlapAngleV2.mlx
  note: Flap Command Angle to Steps
  note: Stepper Angle to Flap Angle
  command (rad) : Inport
  Atan : Trigonometry  Operator=atan2
  Connector Length : Constant  Value=69
  Flap Connector Hinge Offset : Constant  Value=4
  Flap Hinge to Hinge Distance : Constant  Value=41.74793
  Nut Distance at 0 degrees flaps : Constant  Value=107.9382
  Nut Hinge to Flap Hinge Horizontal Distance : Constant  Value=23.48979
  Sqrt : Sqrt
  Square : Math  Operator=square
  Square1 : Math  Operator=square
  Stepper Approximation : Subsystem
  Sum : Sum  Inputs=+|+
  deg2rev : Gain  Gain=1/360
  mm2rad : Subsystem
      settings: PortSchema="{\"entries\":[{\"content\":{\"sides\":[{\"content\":{\"connectorIds\":[\"In1\"]},\"type\":\"ConnectorPlacement.EquallySpacedRectSide\",\"uuid\":\"71648a98-b78c-43f3-816a-917bc6956e0d\"},{\"content\":{\"connectorIds\":[\"Out1\"],\"side\":\"RIGHT\"},\"type\":\"ConnectorPlacement.EquallySpacedRectSide\",\"uuid\":\"f3b64ea6-f0dc-4224-a1ac-a2a818df93ce\"},{\"content\":{\"connectorIds\":[\"In2\",\"In3\",\"In4\",\"In5\",\"In6\"],\"side\":\"TOP\"},\"type\":\"ConnectorPlacement.EquallySpacedRectSide\",\"uuid\":\"ae193476-a4f5-49c0-b052-ecd2bf29d238\"}]},\"type\":\"ConnectorPlacement.EquallySpacedConnector\",\"uuid\":\"a31575f1-a6b5-470b-a3fc-54f09439468e\"}],\"packageUris\":[\"http://schema.mathworks.com/mf0/Connector/R2020b\"],\"version\":\"1.0\"}"
  mm2rev : Gain  Gain=1/2.54
  rad2mm : Subsystem
      settings: PortSchema="{\"entries\":[{\"content\":{\"sides\":[{\"content\":{\"connectorIds\":[\"In1\"]},\"type\":\"ConnectorPlacement.EquallySpacedRectSide\",\"uuid\":\"71648a98-b78c-43f3-816a-917bc6956e0d\"},{\"content\":{\"connectorIds\":[\"Out1\"],\"side\":\"RIGHT\"},\"type\":\"ConnectorPlacement.EquallySpacedRectSide\",\"uuid\":\"f3b64ea6-f0dc-4224-a1ac-a2a818df93ce\"},{\"content\":{\"connectorIds\":[\"In2\",\"In3\",\"In4\",\"In5\",\"In6\"],\"side\":\"TOP\"},\"type\":\"ConnectorPlacement.EquallySpacedRectSide\",\"uuid\":\"ae193476-a4f5-49c0-b052-ecd2bf29d238\"},{\"content\":{\"side\":\"BOTTOM\"},\"type\":\"ConnectorPlacement.EquallySpacedRectSide\",\"uuid\":\"0f3cdbc2-8cff-46b8-9ca1-c72428c01618\"}]},\"type\":\"ConnectorPlacement.EquallySpacedConnector\",\"uuid\":\"a31575f1-a6b5-470b-a3fc-54f09439468e\"}],\"packageUris\":[\"http://schema.mathworks.com/mf0/Connector/R2020b\"],\"version\":\"1.0\"}"
  rev2deg : Gain  Gain=360
  rev2mm : Gain  Gain=2.54
  response (rad) : Outport
  wires:
  deg2rev/1 -> rev2mm/1
  rev2mm/1 -> mm2rad/1(mm)
  ? -> deg2rev/1
  mm2rad/1(rad) -> response (rad)/1
  command (rad)/1 -> rad2mm/1(rad)
  rad2mm/1(mm) -> mm2rev/1
  mm2rev/1 -> rev2deg/1
  Connector Length/1 -> rad2mm/3(Z), mm2rad/3(Z)  "Z"
  Flap Connector Hinge Offset/1 -> Atan/1, Square1/1  "Y"
  Flap Hinge to Hinge Distance/1 -> Square/1, Atan/2  "X"
  Nut Hinge to Flap Hinge Horizontal Distance/1 -> mm2rad/2(B), rad2mm/2(B)  "B"
  Sum/1 -> Sqrt/1
  Square1/1 -> Sum/1
  Square/1 -> Sum/2
  Sqrt/1 -> rad2mm/5(W), mm2rad/5(W)  "W"
  Atan/1 -> mm2rad/4(gamma), rad2mm/4(gamma)  "gamma"
  Nut Distance at 0 degrees flaps/1 -> rad2mm/6(A_0), mm2rad/6(A_0)  "A_0"
  rev2deg/1 -> ?

== system FlapDuuuuuragControlSimulatorForFriends/User Parameters/Stepper Approximation ==
  theta_desired (deg) : Inport
  Initial State Setter : UnitDelay  SampleTime=-1  HasFrameUpgradeWarning=on
  Scope : Scope  NumInputPorts=2
  deg/s limiter : RateLimiter  RisingSlewLimit=4500  FallingSlewLimit=-4500  SampleTimeMode=inherited
  theta_actual (deg) : Outport
  wires:
  Initial State Setter/1 -> deg/s limiter/1, Scope/1  "desired"
  deg/s limiter/1 -> theta_actual (deg)/1, Scope/2  "actual"
  theta_desired (deg)/1 -> Initial State Setter/1  "desired"

== system FlapDuuuuuragControlSimulatorForFriends/User Parameters/Wind Conditions ==
  Constant Wind (Cartesian) : Subsystem  VariantControl=Wind Conditions1
  Wind & Gust (Polar) : Subsystem  VariantControl=Wind Conditions
  Wind (m/s) : Outport
  Out2 : Outport  Port=2

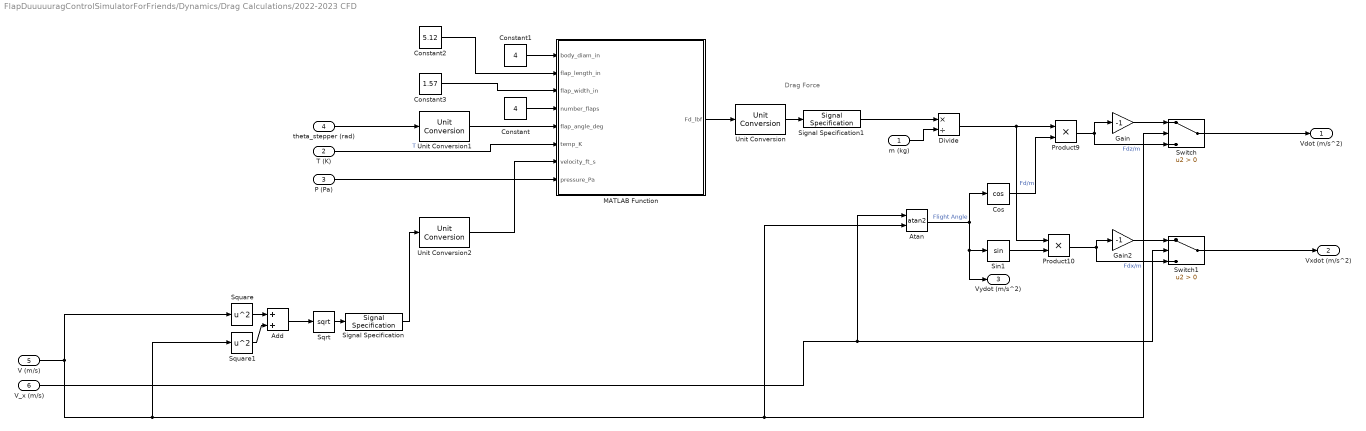
== system FlapDuuuuuragControlSimulatorForFriends/Dynamics/Drag Calculations/2022-2023 CFD ==
  note: Drag Force
  m (kg) : Inport  Unit=kg
  T (K) : Inport  Port=2  Unit=K
  P (Pa) : Inport  Port=3  Unit=Pa
  theta_stepper (rad) : Inport  Port=4  Unit=rad
  V (m/s) : Inport  Port=5  Unit=m/s
  V_x (m/s) : Inport  Port=6  Unit=m/s
  Add : Sum
  Atan : Trigonometry  Operator=atan2
  Constant : Constant  Value=4
  Constant1 : Constant  Value=4
  Constant2 : Constant  Value=5.12
  Constant3 : Constant  Value=1.57
  Cos : Trigonometry  Operator=cos
  Divide : Product  Inputs=*/
  Gain : Gain  Gain=-1
  Gain2 : Gain  Gain=-1
  MATLAB Function : MATLAB Function  TreatAsAtomicUnit=on
  Product10 : Product
  Product9 : Product
  Signal Specification : SignalSpecification  Unit=m/s
  Signal Specification1 : SignalSpecification  Unit=N
  Sin1 : Trigonometry
  Sqrt : Sqrt
  Square : Math  Operator=square
  Square1 : Math  Operator=square
  Switch : Switch  Criteria=u2 > Threshold  SaturateOnIntegerOverflow=off  InputSameDT=off
  Switch1 : Switch  Criteria=u2 > Threshold  SaturateOnIntegerOverflow=off  InputSameDT=off
  Unit Conversion : UnitConversion
  Unit Conversion1 : UnitConversion
  Unit Conversion2 : UnitConversion
  Vdot (m/s^2) : Outport  Unit=m/s^2
  Vxdot (m/s^2) : Outport  Port=2  Unit=m/s^2
  Vydot (m/s^2) : Outport  Port=3
  wires:
  Cos/1 -> Product9/2
  V_x (m/s)/1 -> Switch1/2, Atan/1
  Atan/1 -> Cos/1, Vydot (m/s^2)/1, Sin1/1  "Flight Angle"
  Gain2/1 -> Switch1/1
  Product9/1 -> Gain/1, Switch/3  "Fdz/m"
  Switch1/1 -> Vxdot (m/s^2)/1
  Product10/1 -> Switch1/3, Gain2/1  "Fdx/m"
  Gain/1 -> Switch/1
  Switch/1 -> Vdot (m/s^2)/1
  V (m/s)/1 -> Square1/1, Atan/2, Switch/2, Square/1
  Sin1/1 -> Product10/2
  Divide/1 -> Product10/1, Product9/1  "Fd/m"
  MATLAB Function/1(Fd_lbf) -> Unit Conversion/1
  m (kg)/1 -> Divide/2
  P (Pa)/1 -> MATLAB Function/8(pressure_Pa)
  theta_stepper (rad)/1 -> Unit Conversion1/1
  Unit Conversion1/1 -> MATLAB Function/5(flap_angle_deg)
  T (K)/1 -> MATLAB Function/6(temp_K)  "T"
  Square/1 -> Add/1
  Square1/1 -> Add/2
  Add/1 -> Sqrt/1
  Signal Specification/1 -> Unit Conversion2/1
  Unit Conversion2/1 -> MATLAB Function/7(velocity_ft_s)
  Constant/1 -> MATLAB Function/4(number_flaps)
  Constant3/1 -> MATLAB Function/3(flap_width_in)
  Constant2/1 -> MATLAB Function/2(flap_length_in)
  Constant1/1 -> MATLAB Function/1(body_diam_in)
  Sqrt/1 -> Signal Specification/1
  Unit Conversion/1 -> Signal Specification1/1
  Signal Specification1/1 -> Divide/1

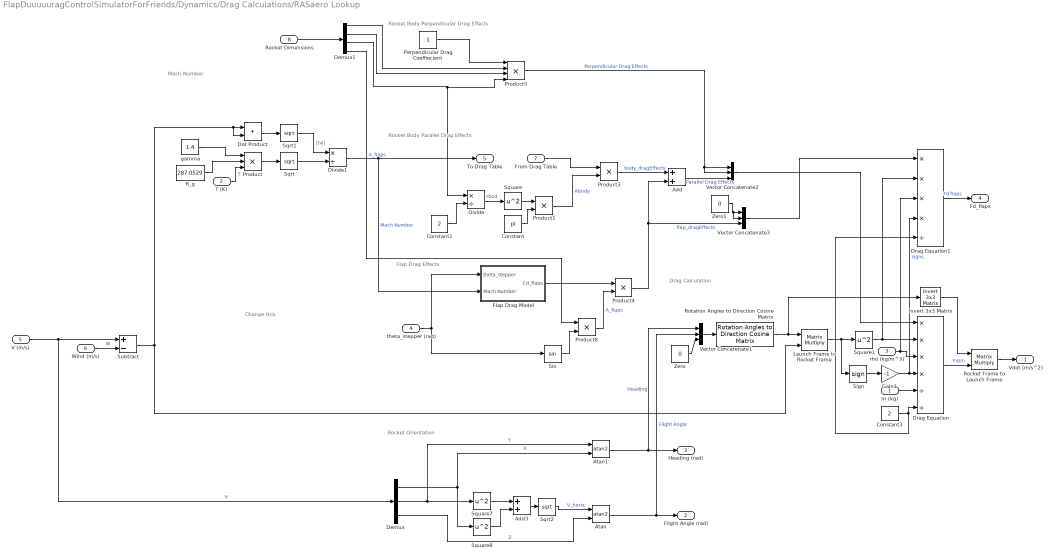
== system FlapDuuuuuragControlSimulatorForFriends/Dynamics/Drag Calculations/RASaero Lookup ==
  note: Change this
  note: Drag Calculation
  note: Rocket Body Perpendicular Drag Effects
  note: Rocket Orientation
  note: Rocket Body Parallel Drag Effects
  note: Flap Drag Effects
  note: Mach Number
  m (kg) : Inport
  T (K) : Inport  Port=2  PortDimensions=1
  rho (kg/m^3) : Inport  Port=3  PortDimensions=1
  theta_stepper (rad) : Inport  Port=4
  V (m/s) : Inport  Port=5
  Wind (m/s) : Inport  Port=6
  From Drag Table : Inport  Port=7
  Rocket Dimensions : Inport  Port=8
  Add : Sum
  Add3 : Sum
  Atan : Trigonometry  Operator=atan2
  Atan1 : Trigonometry  Operator=atan2
  Constant : Constant  Value=pi
  Constant1 : Constant  Value=2
  Constant3 : Constant  Value=2
  Demux : Demux  Outputs=3
  Demux1 : Demux
  Divide : Product  Inputs=*/
  Divide1 : Product  Inputs=*/
  Dot Product : DotProduct  OutDataTypeStr=Inherit: Inherit via internal rule
  Drag Equation : Product  Inputs=****//
  Drag Equation1 : Product  Inputs=****/
  Flap Drag Model : Subsystem
  Gain1 : Gain  Gain=-1
  Invert 3x3 Matrix : aerolibutil/Invert  3x3 Matrix
  Launch Frame to Rocket Frame : Product  Multiplication=Matrix(*)
  Perpendicular Drag Coeffiecient : Constant
  Product : Product  Inputs=3
  Product{1,3..4,8} (4 alike) : Product
  Product5 : Product  Inputs=4
  R_g : Constant  Value=287.0529
  Rocket Frame to Launch Frame : Product  Multiplication=Matrix(*)
  Rotation Angles to Direction Cosine Matrix : sharedtransform/Rotation Angles to Direction Cosine Matrix  rotationOrder=ZYX  aMode=aMode
  Sign : Signum  ZeroCross=off
  Sin : Trigonometry
  Sqrt : Sqrt
  Sqrt1 : Sqrt
  Sqrt2 : Sqrt
  Square{,1,7..8} (4 alike) : Math  Operator=square
  Subtract : Sum  Inputs=+-
  Vector Concatenate1 : Concatenate  NumInputs=3
  Vector Concatenate2 : Concatenate  NumInputs=3
  Vector Concatenate3 : Concatenate  NumInputs=3
  Zero : Constant  Value=0  OutDataTypeStr=Inherit: Inherit via back propagation
  Zero1 : Constant  Value=0  OutDataTypeStr=Inherit: Inherit via back propagation
  gamma : Constant  Value=1.4
  Vdot (m/s^2) : Outport
  Flight Angle (rad) : Outport  Port=2
  Heading (rad) : Outport  Port=3
  Fd_flaps : Outport  Port=4
  To Drag Table : Outport  Port=5
  wires:
  Constant1/1 -> Divide/2
  Atan/1 -> Vector Concatenate1/2, Flight Angle (rad)/1  "Flight Angle"
  Sin/1 -> Product8/2
  Add/1 -> Vector Concatenate2/3  "Parallel Drag Effects"
  theta_stepper (rad)/1 -> Sin/1, Flap Drag Model/1(theta_stepper)
  Demux1/3 -> Divide/1, Product5/4
  m (kg)/1 -> Drag Equation/5
  Drag Equation/1 -> Rocket Frame to Launch Frame/2  "Fd/m"
  Divide/1 -> Square/1  "rbod"
  Product1/1 -> Product3/2  "Abody"
  Product3/1 -> Add/1  "body_dragEffects"
  Product8/1 -> Product4/2  "A_flaps"
  Square/1 -> Product1/1
  Constant/1 -> Product1/2
  Flap Drag Model/1(Cd_flaps) -> Product4/1
  Product4/1 -> Vector Concatenate3/3, Add/2  "flap_dragEffects"
  Constant3/1 -> Drag Equation/6, Drag Equation1/5
  Demux1/4 -> Product8/1  "A_flaps"
  Divide1/1 -> To Drag Table/1, Flap Drag Model/2(Mach Number)  "Mach Number"
  Product/1 -> Sqrt/1
  Sqrt/1 -> Divide1/2
  Sqrt1/1 -> Divide1/1  "||v||"
  R_g/1 -> Product/2
  gamma/1 -> Product/1
  T (K)/1 -> Product/3  "T"
  Square7/1 -> Add3/1
  Square8/1 -> Add3/2
  Add3/1 -> Sqrt2/1
  Sqrt2/1 -> Atan/1  "V_horiz"
  Atan1/1 -> Heading (rad)/1, Vector Concatenate1/1  "Heading"
  rho (kg/m^3)/1 -> Drag Equation1/3, Drag Equation/3
  Rocket Frame to Launch Frame/1 -> Vdot (m/s^2)/1
  V (m/s)/1 -> Demux/1, Subtract/1  "V"
  Wind (m/s)/1 -> Subtract/2  "W"
  Demux/3 -> Atan/2  "Z"
  Demux/1 -> Square8/1, Atan1/2  "X"
  Demux/2 -> Square7/1, Atan1/1  "Y"
  Dot Product/1 -> Sqrt1/1
  Vector Concatenate1/1 -> Rotation Angles to Direction Cosine Matrix/1
  Zero/1 -> Vector Concatenate1/3
  Rotation Angles to Direction Cosine Matrix/1 -> Launch Frame to Rocket Frame/1, Invert 3x3 Matrix/1
  Launch Frame to Rocket Frame/1 -> Sign/1, Square1/1
  Square1/1 -> Drag Equation1/2, Drag Equation/2
  Perpendicular Drag Coeffiecient/1 -> Product5/1
  Demux1/1 -> Product5/2
  Demux1/2 -> Product5/3
  Product5/1 -> Vector Concatenate2/1, Vector Concatenate2/2  "Perpendicular Drag Effects"
  Vector Concatenate2/1 -> Drag Equation/1
  Invert 3x3 Matrix/1 -> Rocket Frame to Launch Frame/1
  Subtract/1 -> Launch Frame to Rocket Frame/2, Dot Product/2, Dot Product/1
  Sign/1 -> Gain1/1
  Gain1/1 -> Drag Equation1/4, Drag Equation/4  "signs"
  Zero1/1 -> Vector Concatenate3/2, Vector Concatenate3/1
  Vector Concatenate3/1 -> Drag Equation1/1
  Drag Equation1/1 -> Fd_flaps/1  "Fd flaps"
  From Drag Table/1 -> Product3/1
  Rocket Dimensions/1 -> Demux1/1

== system FlapDuuuuuragControlSimulatorForFriends/User Parameters/Control System/Controller (coppied from L2) ==
  In1 : Inport
  Input : Inport  Port=2
  Double Integrator : Subsystem  VariantControl=false
  Gain Scheduling : Subsystem  VariantControl=false
  PID : Subsystem  VariantControl=true
  Shennanigans : Subsystem  VariantControl=false
  Shennanigans Part 2 : Subsystem  VariantControl=false
  Out1 : Outport

== system FlapDuuuuuragControlSimulatorForFriends/User Parameters/Control System/Projection ==
  h : Inport
  v : Inport  Port=2
  Add : Sum
  Constant : Constant  Value=2
  Divide : Product  Inputs=*/
  Product : Product  Inputs=*/
  Product1 : Product
  Square : Math  Operator=square
  g : Constant  Value=9.8
  h_prediction : Outport
  wires:
  Add/1 -> Divide/1  "Pe_final"
  v/1 -> Square/1
  Product/1 -> Add/1  "Ke"
  Constant/1 -> Product/2
  Product1/1 -> Add/2  "Pe"
  Square/1 -> Product/1
  h/1 -> Product1/1
  g/1 -> Divide/2, Product1/2
  Divide/1 -> h_prediction/1

== system FlapDuuuuuragControlSimulatorForFriends/User Parameters/Flap Response/Stepper Approximation ==
  theta_desired (deg) : Inport
  Initial State Setter : UnitDelay  SampleTime=-1  HasFrameUpgradeWarning=on
  Scope : Scope  NumInputPorts=2
  deg/s limiter : RateLimiter  RisingSlewLimit=4500  FallingSlewLimit=-4500  SampleTimeMode=inherited
  theta_actual (deg) : Outport
  wires:
  Initial State Setter/1 -> deg/s limiter/1, Scope/1  "desired"
  deg/s limiter/1 -> theta_actual (deg)/1, Scope/2  "actual"
  theta_desired (deg)/1 -> Initial State Setter/1  "desired"

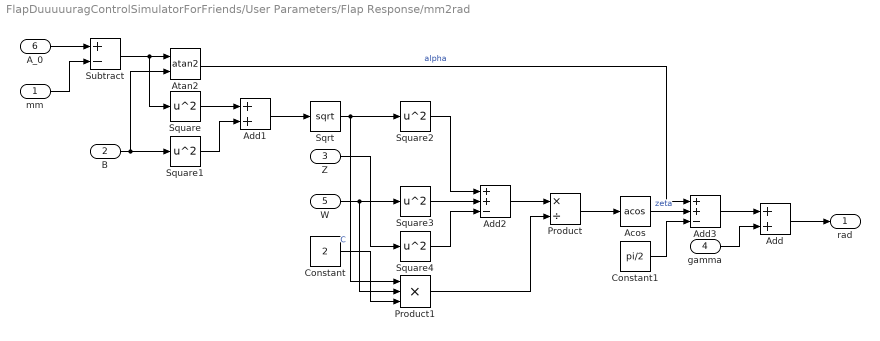
== system FlapDuuuuuragControlSimulatorForFriends/User Parameters/Flap Response/mm2rad ==
  mm : Inport
  B : Inport  Port=2
  Z : Inport  Port=3
  gamma : Inport  Port=4
  W : Inport  Port=5
  A_0 : Inport  Port=6
  Acos : Trigonometry  Operator=acos
  Add : Sum
  Add1 : Sum
  Add2 : Sum  Inputs=++-
  Add3 : Sum  Inputs=++-
  Atan2 : Trigonometry  Operator=atan2
  Constant : Constant  Value=2
  Constant1 : Constant  Value=pi/2
  Product : Product  Inputs=*/
  Product1 : Product  Inputs=3
  Sqrt : Sqrt
  Square{,1..4} (5 alike) : Math  Operator=square
  Subtract : Sum  Inputs=+-
  rad : Outport
  wires:
  Square4/1 -> Add2/3
  Atan2/1 -> Add3/1  "alpha"
  Add/1 -> rad/1
  A_0/1 -> Subtract/1
  Add1/1 -> Sqrt/1
  Add2/1 -> Product/1
  Square3/1 -> Add2/2
  mm/1 -> Subtract/2
  Acos/1 -> Add3/2  "zeta"
  Subtract/1 -> Square/1, Atan2/1
  B/1 -> Square1/1, Atan2/2
  Square/1 -> Add1/1
  gamma/1 -> Add/2
  Square2/1 -> Add2/1
  Square1/1 -> Add1/2
  Sqrt/1 -> Product1/1, Square2/1  "C"
  W/1 -> Product1/2, Square3/1
  Z/1 -> Square4/1
  Constant/1 -> Product1/3
  Product1/1 -> Product/2
  Product/1 -> Acos/1
  Constant1/1 -> Add3/3
  Add3/1 -> Add/1

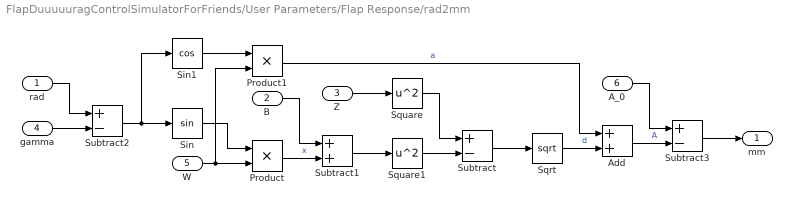
== system FlapDuuuuuragControlSimulatorForFriends/User Parameters/Flap Response/rad2mm ==
  rad : Inport
  B : Inport  Port=2
  Z : Inport  Port=3
  gamma : Inport  Port=4
  W : Inport  Port=5
  A_0 : Inport  Port=6
  Add : Sum
  Product : Product
  Product1 : Product
  Sin : Trigonometry
  Sin1 : Trigonometry  Operator=cos
  Sqrt : Sqrt
  Square : Math  Operator=square
  Square1 : Math  Operator=square
  Subtract : Sum  Inputs=+-
  Subtract1 : Sum
  Subtract2 : Sum  Inputs=+-
  Subtract3 : Sum  Inputs=+-
  mm : Outport
  wires:
  W/1 -> Product1/2, Product/2
  rad/1 -> Subtract2/1
  Subtract2/1 -> Sin1/1, Sin/1
  B/1 -> Subtract1/1
  Product1/1 -> Add/1  "a"
  gamma/1 -> Subtract2/2
  Sin1/1 -> Product1/1
  Sin/1 -> Product/1
  Product/1 -> Subtract1/2  "x"
  Z/1 -> Square/1
  Subtract1/1 -> Square1/1
  Square/1 -> Subtract/1
  Square1/1 -> Subtract/2
  Subtract/1 -> Sqrt/1
  Sqrt/1 -> Add/2  "d"
  A_0/1 -> Subtract3/1
  Add/1 -> Subtract3/2  "A"
  Subtract3/1 -> mm/1

== system FlapDuuuuuragControlSimulatorForFriends/User Parameters/Wind Conditions/Constant Wind (Cartesian) ==
  Vector Concatenate : Concatenate  NumInputs=3
  Wind_X (m/s) : Constant  Commented=on  Value=4
  Wind_Y (m/s) : Constant  Commented=on  Value=4
  Wind_Z (m/s) : Constant  Commented=on  Value=0
  Wind (m/s) : Outport
  wires:
  Wind_Z (m/s)/1 -> Vector Concatenate/3
  Wind_X (m/s)/1 -> Vector Concatenate/1
  Wind_Y (m/s)/1 -> Vector Concatenate/2
  Vector Concatenate/1 -> Wind (m/s)/1

== system FlapDuuuuuragControlSimulatorForFriends/User Parameters/Wind Conditions/Wind & Gust (Polar) ==
  note: The wind shear model can help give you an idea of windspeed at various heights above ground level based solely one the measurement at ground level. I'm unsure how it changes by direction. The DCM deals with ECI and FE coordinate systems. It may be possible to ignore these?
  Cos : Trigonometry  Operator=cos
  Discrete Wind Gust Model : aerolibwind2/Discrete Wind Gust Model  Commented=on  units=Metric (MKS)  Gx=on  Gy=on  Gz=on  t_0=5  d_m=[120 120 80]  v_m=[3.5 3.5 3.0]
  Product : Product
  Product1 : Product
  Sin : Trigonometry
  Sum : Sum  Inputs=|++
  Vector Concatenate : Concatenate  NumInputs=3
  Wind Gust(s) : DiscretePulseGenerator  PulseType=Time based  Amplitude=0  Period=20  PulseWidth=25
  Wind Shear Model : aerolibwind2/Wind Shear Model  Commented=on  units=Metric (MKS)  phase=Other  W_20=15  Wdeg=0
  Wind_Z (m/s)1 : Constant  Value=wind_Z
  Wind_direction (rad) : Constant  Value=wind_direction
  Wind_speed (m/s) : Constant  Value=wind_speed
  Wind (m/s) : Outport
  wires:
  Sum/1 -> Product/1, Product1/1
  Cos/1 -> Product/2
  Product1/1 -> Vector Concatenate/2  "Wy"
  Sin/1 -> Product1/2
  Wind_direction (rad)/1 -> Cos/1, Sin/1
  Wind_speed (m/s)/1 -> Sum/2
  Wind Gust(s)/1 -> Sum/1
  Product/1 -> Vector Concatenate/1  "Wx"
  Wind_Z (m/s)1/1 -> Vector Concatenate/3
  Vector Concatenate/1 -> Wind (m/s)/1

== system FlapDuuuuuragControlSimulatorForFriends/Dynamics/Drag Calculations/RASaero Lookup/Flap Drag Model ==
  note: TODO: Vary the max Cd with Mach number
  theta_stepper : Inport
  Mach Number : Inport  Port=2
  Cd_full_flaps : Constant
  Divide1 : Product  Inputs=**
  Sin : Trigonometry
  Cd_flaps : Outport
  wires:
  theta_stepper/1 -> Sin/1
  Divide1/1 -> Cd_flaps/1  "Cd_flaps"
  Cd_full_flaps/1 -> Divide1/1
  Sin/1 -> Divide1/2
